simulink model "GNa_model"  (Simulink 3.00)
settings: Solver=ode45  StartTime=0.0  StopTime=20  FixedStep=0.01  RelTol=1e-3
settings Model: Creator=angel  LastModifiedBy=angel

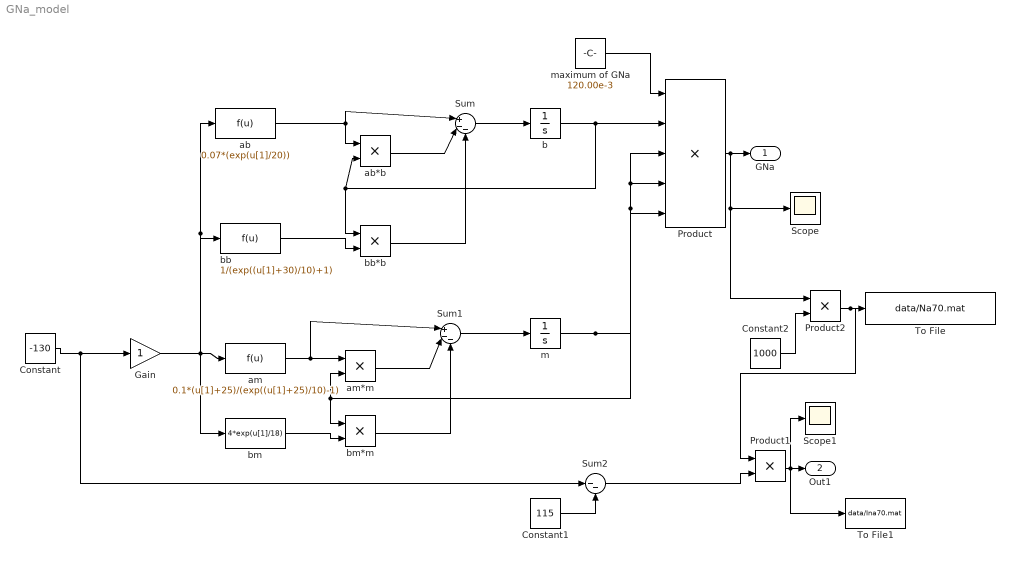
== system GNa_model ==
  Constant : Constant  Value=-130
  Constant1 : Constant  Value=115
  Constant2 : Constant  Value=1000
  Gain : Gain  Gain=1  SaturateOnIntegerOverflow=on
  Product : Product  Inputs=5  SaturateOnIntegerOverflow=on
  Product1 : Product  Inputs=2  SaturateOnIntegerOverflow=on
  Product2 : Product  Inputs=2  SaturateOnIntegerOverflow=on
  Scope : Scope
      settings: TimeRange=auto  YMin=-5  YMax=5  SaveToWorkspace=off  SaveName=ScopeData
  Scope1 : Scope
      settings: TimeRange=auto  YMin=-5  YMax=5  SaveToWorkspace=off  SaveName=ScopeData
  Sum : Sum  Inputs=|+--  SaturateOnIntegerOverflow=on
  Sum1 : Sum  Inputs=|+--  SaturateOnIntegerOverflow=on
  Sum2 : Sum  Inputs=|--  SaturateOnIntegerOverflow=on
  To File : ToFile  Filename=data/Na70.mat  MatrixName=Gna  SampleTime=-1
  To File1 : ToFile  Filename=data/Ina70.mat  MatrixName=Ina  SampleTime=-1
  ab : Fcn  Expr=0.07*(exp(u[1]/20))
  ab*b : Product  Inputs=2  SaturateOnIntegerOverflow=on
  am : Fcn  Expr=0.1*(u[1]+25)/(exp((u[1]+25)/10)-1)
  am*m : Product  Inputs=2  SaturateOnIntegerOverflow=on
  b : Integrator  ExternalReset=none  InitialConditionSource=internal  InitialCondition=0.59615  LimitOutput=off  UpperSaturationLimit=inf  LowerSaturationLimit=-inf  ShowSaturationPort=off  ShowStatePort=off  AbsoluteTolerance=auto
  bb : Fcn  Expr=1/(exp((u[1]+30)/10)+1)
  bb*b : Product  Inputs=2  SaturateOnIntegerOverflow=on
  bm : Fcn  Expr=4*exp(u[1]/18)
  bm*m : Product  Inputs=2  SaturateOnIntegerOverflow=on
  m : Integrator  ExternalReset=none  InitialConditionSource=internal  InitialCondition=0.05294  LimitOutput=off  UpperSaturationLimit=inf  LowerSaturationLimit=-inf  ShowSaturationPort=off  ShowStatePort=off  AbsoluteTolerance=auto
  maximum of GNa : Constant  Value=120.00e-3
  GNa : Outport  Port=1
  Out1 : Outport  Port=2
  wires:
  bb/1 -> bb*b/2
  ab/1 -> ab*b/1, Sum/1
  ab*b/1 -> Sum/2
  bb*b/1 -> Sum/3
  bm/1 -> bm*m/2
  am*m/1 -> Sum1/2
  bm*m/1 -> Sum1/3
  am/1 -> am*m/1, Sum1/1
  Sum/1 -> b/1
  b/1 -> ab*b/2, bb*b/1, Product/2
  m/1 -> am*m/2, bm*m/1, Product/3, Product/4, Product/5
  maximum of GNa/1 -> Product/1
  Sum1/1 -> m/1
  Gain/1 -> am/1, ab/1, bb/1, bm/1
  Constant/1 -> Gain/1, Sum2/1
  Constant1/1 -> Sum2/2
  Sum2/1 -> Product1/2
  Product/1 -> GNa/1, Scope/1, Product2/1
  Product1/1 -> Scope1/1, Out1/1, To File1/1
  Constant2/1 -> Product2/2
  Product2/1 -> To File/1, Product1/1
